simulink model "HIL_PLANT_r2025a"  (R2025a)
settings: Solver=FixedStepAuto  StartTime=0.0  StopTime=inf  MaxStep=1e-2  RelTol=1e-3  AbsTol=1e-3  EnableMultiTasking=on
undefined symbols (not defined in the file): IO334, IO336, pull, up
libraries: fl_lib x12, nesl_utility x4, speedgoatlib_fpga_analog_io x3, speedgoatlib_fpga x1
CloseFcn:
  | try,close(h1_PermanentMagnetDCMotor),end
  | clear h1_PermanentMagnetDCMotor
  | 
  | clear simlog_PermanentMagnetDCMotor
Description:
  | Permanent Magnet DC Motor
settings Model: Creator=The MathWorks, Inc.  LastModifiedBy=AEDemo
settings SolverCC: AutoScaleAbsTol=off  ConcurrentTasks=on  AlgebraicLoopSolver=TrustRegion  PositivePriorityOrder=on
settings DataIOCC: LimitDataPoints=on  SaveFormat=Array  ReturnWorkspaceOutputs=off
settings OptimizationCC: BlockReduction=off  OptimizeBlockIOStorage=off  ReuseModelBlockBuffer=off  InitFltsAndDblsToZero=on
settings DebuggingCC: SolverPrmCheckMsg=warning  TasksWithSamePriorityMsg=none  UnconnectedInputMsg=warning  UnconnectedOutputMsg=warning  UnconnectedLineMsg=warning  AllowSymbolicDim=off  PregeneratedLibrarySubsystemCodeDiagnostic=none  SFUnexpectedBacktrackingDiag=warning  SFNoUnconditionalDefaultTransitionDiag=warning  SFExecutionAtInitializationDiag=none  ArithmeticOperatorsInVariantConditions=warning
settings HardwareCC: ProdBitPerLong=64.0  ProdLongLongMode=on  ProdHWDeviceType=Intel->x86-64 (Linux 64)  TargetLongLongMode=on
settings ModelReferenceCC: EnableRefExpFcnMdlSchedulingChecks=on  PropagateSignalLabelsOutOfModel=off
settings SFSimCC: SimUseLocalCustomCode=off  CustomCodeUndefinedFunction=UseInterfaceOnly
settings RTWCC: SystemTargetFile=speedgoat.tlc  TemplateMakefile=slrealtime_default_tmf  RTWUseLocalCustomCode=off  Toolchain=Simulink Real-Time Toolchain  BuildConfiguration=Faster Runs  CodeExecutionProfiling=on  TargetLang=C++  GPUComputeCapability=3.5  DLArmComputeVersion=19.05  Description=Speedgoat Real-Time Target Machine
settings CodeAppCC: StateflowObjectComments=on
settings SimulinkRealTimeTargetCC: SLRTFileLogMaxRuns=1.0  ExtModeMaxTrigDuration=10.0  ExtModeStaticAllocSize=1000000.0  ExtModeTransport=0.0  MultiwordLength=2048.0  DynamicStringBufferSize=256.0  PreserveMATLABNamespacesInGeneratedCode=on  SubcomponentCodeInterfacePackaging=Reusable function  MATLABClassNameForMDSCustomization=Simulink.SoftwareTarget.GRTCustomization  InstructionSetFMA=off  LogToMDFFile=off
settings ConfigComp: CovMetricSettings=dw  CovSaveCumulativeToWorkspaceVar=on  CovSaveSingleToWorkspaceVar=on  CovExternalEMLEnable=off  CovSFcnEnable=off
settings SimscapeCC: SimscapeLogType=all  SimscapeLogSimulationStatistics=on  SimscapeLogName=simlog_PermanentMagnetDCMotor  SimscapeLogDataHistory=10000.0

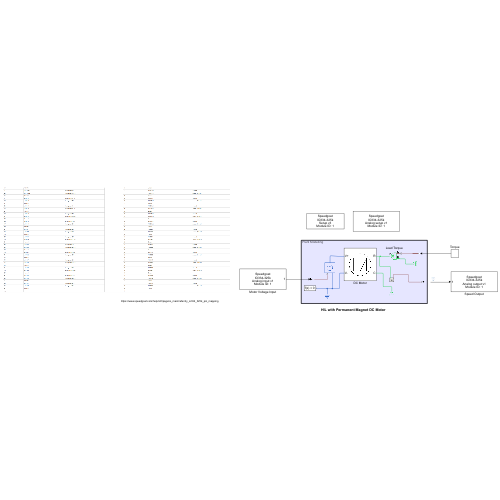
[thumbnail: Simulink's stored preview of the top-level diagram]
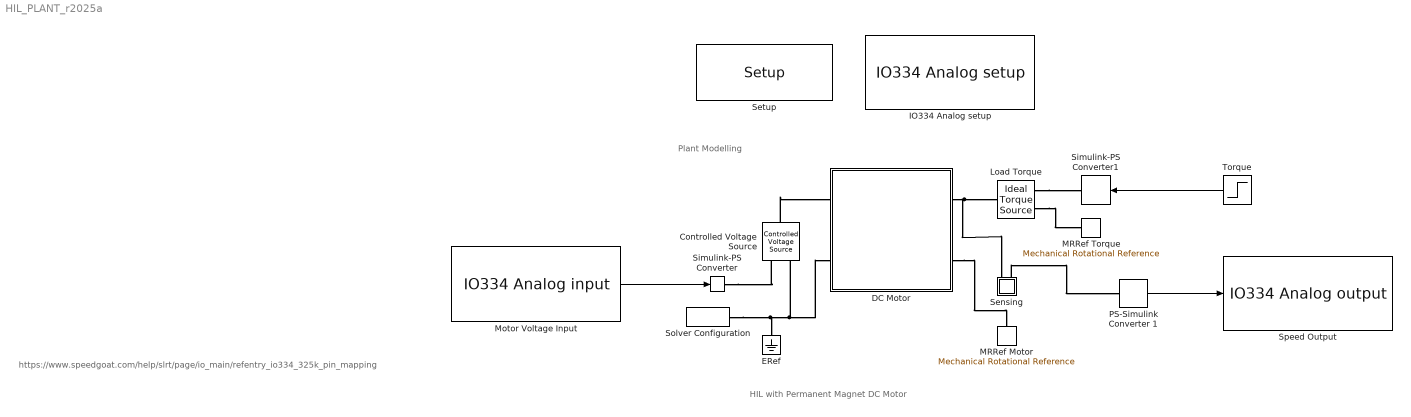
== system HIL_PLANT_r2025a ==
  note: https://www.speedgoat.com/help/slrt/page/io_main/refentry_io334_325k_pin_mapping
  note: Plant Modelling
  note: HIL with Permanent Magnet DC Motor
  Controlled Voltage Source : fl_lib/Electrical/Electrical Sources/Controlled Voltage Source
  DC Motor : Subsystem  Tag=PublishSubsystem
      mask Display:
      | % Circle, in/out, and 'M'
      | image('PermanentMagnetDCMotorMaskIcon.png');
      | 
      | % % Circle
      | % plot(sin(0:0.1:2.2*pi)*0.9,cos(0:0.1:2.2*pi)*0.9);
      | %
      | % % In/out
      | % plot([-1.3 -0.9],[0 0]);
      | % plot([1.3 0.9],[0 0]);
      | %
      | % % 'M'
      | % plot([0.5 0.5],[-0.5 0.5]);
      | % plot([-0.5 -0.5],[-0.5 0.5]);
      | % plot([0.5 0],[0.5 -0.5]);
      | % plot([-0.5 0],[0.5 -0.5]);
      | 
      | % Plot points to set plot range
      | color('white');plot(1.5,1.5);plot(-1.5,-1.5)
      | color('black');
      | 
      | port_label('RConn',1,'R');
      | port_label('RConn',2,'C');
      | port_label('LConn',1,'V+');
      | port_label('LConn',2,'V-');
  ERef : fl_lib/Electrical/Electrical Elements/Electrical Reference
  IO334 Analog setup : speedgoatlib_fpga_analog_io/IO334/IO334 Analog setup  id=1  parEnableCodeModule1=off  parEnableCodeModule2=off  parEnableCodeModule3=off  parEnableCodeModule4=off  parEnableCodeModule5=off  parEnableCodeModule6=off  parEnableCodeModule7=off  parEnableCodeModule8=off  parAdcEnableIndividualTrigger=off  parAdcDisableSampleRead=off  parAdcTriggerMode1=Model Step  parAdcSampleRate1=1e5  parAdcDioTriggerChannel1=1  parAdcInternalTrigger1=<empty>  parAdcOversampling1=None  parAdcTriggerMode2=Model Step  parAdcSampleRate2=1e5  parAdcDioTriggerChannel2=1  parAdcInternalTrigger2=<empty>  parAdcOversampling2=None  parAdcTriggerMode3=Model Step  parAdcSampleRate3=1e5  parAdcDioTriggerChannel3=1  parAdcInternalTrigger3=<empty>  parAdcOversampling3=None  parAdcTriggerMode4=Model Step  parAdcSampleRate4=1e5  parAdcDioTriggerChannel4=1  parAdcInternalTrigger4=<empty>  parAdcOversampling4=None  parAdcTriggerMode5=Model Step  parAdcSampleRate5=1e5  parAdcDioTriggerChannel5=1  parAdcInternalTrigger5=<empty>  parAdcOversampling5=None  parAdcTriggerMode6=Model Step  parAdcSampleRate6=1e5  parAdcDioTriggerChannel6=1  parAdcInternalTrigger6=<empty>  parAdcOversampling6=None  parAdcTriggerMode7=Model Step  parAdcSampleRate7=1e5  parAdcDioTriggerChannel7=1  parAdcInternalTrigger7=<empty>  parAdcOversampling7=None  parAdcTriggerMode8=Model Step  parAdcSampleRate8=1e5  parAdcDioTriggerChannel8=1  parAdcInternalTrigger8=<empty>  parAdcOversampling8=None  parAdcReadPrevValueIndividualTrigger=off  parAdcEnableFrame=off  parAdcTriggerMode=I/O Module Clock  parAdcReadPrevValue=on  parAdcSampleRate=100e3  parAdcDioTriggerChannel=1  parAdcInternalTrigger=<empty>  parAdcOversampling=None  parAdcTriggerResolution=1e-08  parAdcSampleRateFrame=1e5  parAdcFrameSize=100  parAdcSampleTime=-1  parDacTriggerMode=Model Step  parDacInternalTrigger=<empty>  parDacDioTriggerChannel=1  parDacEnableFrame=on  parDacFifoThreshold=100  parDacTriggerResolution=1e-08  parDacSampleRate=1e6  parDacFrameSize=1000  parDacSampleTime=-1  parAdcChannel1=on  parAdcChannel2=off  parAdcChannel3=off  parAdcChannel4=off  parAdcChannel5=off  parAdcChannel6=off  parAdcChannel7=off  parAdcChannel8=off  parAdcChannel9=off  parAdcChannel10=off  parAdcChannel11=off  parAdcChannel12=off  parAdcChannel13=off  parAdcChannel14=off  parAdcChannel15=off  parAdcChannel16=off  parAdcAutoCorrection=on  parDacChannel1=on  parDacChannel2=off  parDacChannel3=off  parDacChannel4=off  parDacChannel5=off  parDacChannel6=off  parDacChannel7=off  parDacChannel8=off  parDacChannel9=off  parDacChannel10=off  parDacChannel11=off  parDacChannel12=off  parDacChannel13=off  parDacChannel14=off  parDacChannel15=off  parDacChannel16=off  parDacRange1=+-2.5 V  parDacInitValue1=0  parDacReset1=on  parDacRange2=+-10 V  parDacInitValue2=0  parDacReset2=on  parDacRange3=+-5 V  parDacInitValue3=0  parDacReset3=off  parDacRange4=+-5 V  parDacInitValue4=0  parDacReset4=off  parDacRange5=+-5 V  parDacInitValue5=0  parDacReset5=off  parDacRange6=+-5 V  parDacInitValue6=0  parDacReset6=off  parDacRange7=+-5 V  parDacInitValue7=0  parDacReset7=off  parDacRange8=+-5 V  parDacInitValue8=0  parDacReset8=off  parDacRange9=+-5 V  parDacInitValue9=0  parDacReset9=off  parDacRange10=+-5 V  parDacInitValue10=0  parDacReset10=off  parDacRange11=+-5 V  parDacInitValue11=0  parDacReset11=off  parDacRange12=+-5 V  parDacInitValue12=0  parDacReset12=off  parDacRange13=+-5 V  parDacInitValue13=0  parDacReset13=off  parDacRange14=+-5 V  parDacInitValue14=0  parDacReset14=off  parDacRange15=+-5 V  parDacInitValue15=0  parDacReset15=off  parDacRange16=+-5 V  parDacInitValue16=0  parDacReset16=off  parDacAutoCorrection=on
      settings: SourceProductName=Analog IO
  Load Torque : fl_lib/Mechanical/Mechanical Sources/Ideal Torque Source
  MRRef Motor : fl_lib/Mechanical/Rotational Elements/Mechanical Rotational Reference
  MRRef Torque : fl_lib/Mechanical/Rotational Elements/Mechanical Rotational Reference
  Motor Voltage Input : speedgoatlib_fpga_analog_io/IO334/IO334 Analog input  id=1  parSampleTime=-1  pciSlot=[-1,-1]  parAiChannels=1  parAiChannelsStreamed=1  parAiReadPrevValue=0  parAiEnableFrame=0  parAdcCoupling=[1 1 1 1]  parAdcContSampling=0  parAdcDmaEnable=0  parAdcActiveDmaDevices=[1 1 1 1]  parAiFrameSize=100
      settings: SourceProductName=Analog IO
  PS-Simulink Converter 1 : nesl_utility/PS-Simulink Converter  PhysicalDomain=network_engine_domain  SubClassName=ps_output  LeftPortType=input  RightPortType=output  PseudoPeriodic=off  Frequencies=[]  VectorFormat=1-D array  Unit=rad/s  AffineConversion=off
  Sensing : Subsystem
      mask Display: disp('w');
  Setup : speedgoatlib_fpga/Setup/Setup  Parameter124={}  board=IO334-325k  id=1  pciSlot=-1  device_id=1  bitstreamFilePath=[]  bitstreamFile=Please select...  rearEnb_1=off  rearIO_1=None  rearEnb_2=off  rearIO_2=None  ProgSpiFlash=off  ProgBPIFlash=off  useFpgaDmaController=off  PullRPort15=pull-up 3.3V  PullRPort31=pull-up 3.3V  PullRPort47=pull-up 3.3V  PullRPort63=pull-up 3.3V  diffLineTermination_1=on  diffLineTermination_2=on  diffLineTermination_3=on  diffLineTermination_4=on  diffLineTermination_5=on  diffLineTermination_6=on  diffLineTermination_7=on  diffLineTermination_8=on  diffLineTermination_9=on  diffLineTermination_10=on  diffLineTermination_11=on  diffLineTermination_12=on  diffLineTermination_13=on  diffLineTermination_14=on  diffLineTermination_15=on  diffLineTermination_16=on  diffLineTermination_17=on  diffLineTermination_18=on  diffLineTermination_19=on  diffLineTermination_20=on  diffLineTermination_21=on  diffLineTermination_22=on  diffLineTermination_23=on  diffLineTermination_24=on  diffLineTermination_25=on  diffLineTermination_26=on  diffLineTermination_27=on  diffLineTermination_28=on  diffLineTermination_29=on  diffLineTermination_30=on  diffLineTermination_31=on  diffLineTermination_32=on  Vi_Pull_36x_1=Floating  Vo_36x_1=3.3V  Vi_Pull_36x_2=Floating  Vo_36x_2=3.3V  Vi_Pull_36x_3=Floating  Vo_36x_3=3.3V  Vi_Pull_36x_4=Floating  Vo_36x_4=3.3V  Vi_Pull_36x_5=Floating  Vo_36x_5=3.3V  Vi_Pull_36x_6=Floating  Vo_36x_6=3.3V  Vi_Pull_36x_7=Floating  Vo_36x_7=3.3V  Vi_Pull_36x_8=Floating  Vo_36x_8=3.3V  Vi_Pull_36x_9_16=Floating  Vo_36x_9_16=3.3V  Vi_Pull_36x_17_24=Floating  Vo_36x_17_24=3.3V  Vi_Pull_36x_25_32=Floating  Vo_36x_25_32=3.3V  Vi_Pull_36x_33_40=Floating  Vo_36x_33_40=3.3V  Vi_Pull_36x_41_48=Floating  Vo_36x_41_48=3.3V  Vi_Pull_36x_49_56=Floating  Vo_36x_49_56=3.3V  Vi_Pull_36x_57_64=Floating  Vo_36x_57_64=3.3V  PullRPort0_1=pull-up  VioPort0_1=3.3V  PullRPort1_1=pull-up  VioPort1_1=3.3V  PullRPort2_1=pull-up  VioPort2_1=3.3V  PullRPort3_1=pull-up  VioPort3_1=3.3V  PullRPort4_1=pull-up  VioPort4_1=3.3V  PullRPort5_1=pull-up  VioPort5_1=3.3V  PullRPort6_1=pull-up  VioPort6_1=3.3V  diffLineTermination_rear1_1=on  diffLineTermination_rear1_2=on  diffLineTermination_rear1_3=on  diffLineTermination_rear1_4=on  diffLineTermination_rear1_5=on  diffLineTermination_rear1_6=on  diffLineTermination_rear1_7=on  diffLineTermination_rear1_8=on  PullRPort0_2=pull-up  VioPort0_2=3.3V  PullRPort1_2=pull-up  VioPort1_2=3.3V  PullRPort2_2=pull-up  VioPort2_2=3.3V  PullRPort3_2=pull-up  VioPort3_2=3.3V  PullRPort4_2=pull-up  VioPort4_2=3.3V  PullRPort5_2=pull-up  VioPort5_2=3.3V  PullRPort6_2=pull-up  VioPort6_2=3.3V  diffLineTermination_rear2_1=on  diffLineTermination_rear2_2=on  diffLineTermination_rear2_3=on  diffLineTermination_rear2_4=on  diffLineTermination_rear2_5=on  diffLineTermination_rear2_6=on  diffLineTermination_rear2_7=on  diffLineTermination_rear2_8=on
      settings: SourceProductName=IO3xx
  Simulink-PS Converter : nesl_utility/Simulink-PS Converter  PhysicalDomain=network_engine_domain  SubClassName=ps_input  LeftPortType=input  RightPortType=output  PseudoPeriodic=off  Frequencies=[]  NoiseDistribution=none  NoiseParameters=[]  Unit=V  AffineConversion=off  FilteringAndDerivatives=provide  SimscapeFilterOrder=1  InputFilterTimeConstant=0.001  UdotUserProvided=0
  Simulink-PS Converter1 : nesl_utility/Simulink-PS Converter  PhysicalDomain=network_engine_domain  SubClassName=ps_input  LeftPortType=input  RightPortType=output  PseudoPeriodic=off  Frequencies=[]  NoiseDistribution=none  NoiseParameters=[]  Unit=1  AffineConversion=off  FilteringAndDerivatives=zero  SimscapeFilterOrder=1  InputFilterTimeConstant=.001  UdotUserProvided=0
  Solver Configuration : nesl_utility/Solver Configuration  PhysicalDomain=network_engine_domain  SubClassName=solver  LeftPortType=input  RightPortType=generic  Tones=[]  Harmonics=[]  SimulateNoise=off  Profile=off  UseLocalSampling=off  EnableSwitchedLinearOptims=on  FrequencyDomain=off  UseCCode=off  RelTol=0.001  AbsTol=1e-06  MinStep=1e-09  ToWorkspace=off  RevertToSquareIcSolve=off  NumHomotopyIterations=100  PhasorMode=off  PhasorModeNumHarmonics=1  ConsistencySolver=NEWTON_XTOL_AFTER_FTOL  IndexReductionMethod=DerivativeReplacement  DoDC=off  ResidualTolerance=1e-9  ConsistencyTolSource=GLOBAL  ConsistencyAbsTol=0.001  ConsistencyRelTol=0.001  ConsistencyTolFactor=0.001  UseLocalSolver=off  LocalSolverChoice=NE_BACKWARD_EULER_ADVANCER  ResolveIndetEquations=on  FunctionEvalNumThread=1  LocalSolverSampleTime=.001  DoFixedCost=off  MaxNonlinIter=3  MaxModeIter=2  ComputeImpulses=off  ImpulseIterations=2  LinearAlgebra=auto  LinearAlgebraNumThread=0  EquationFormulation=NE_TIME_EF  DelaysMemoryBudget=1024  AutomaticFiltering=on  FilteringTimeConstant=0.001  PartitionStorageMethod=AS_NEEDED  PartitionMemoryBudget=1024  PartitionMethod=FAST  MultibodyUseLocalSolver=on  MultibodyLocalSolverChoice=ODE1  MultibodyLocalSolverSampleTime=0.001
  Speed Output : speedgoatlib_fpga_analog_io/IO334/IO334 Analog output  id=1  parSampleTime=-1  pciSlot=[-1,-1]  board=IO336-325k  parAoChannels=1  parAoVoltageRange=3  parDacOverRange=[0 0 0 0 0 0 0 0]  parAoInitValues=0  parAoReset=1  parDacSyncOut=1  parAoEnableFrame=0  parDacActiveDmaDevices=[1 1 1 1]  parDacDmaLatency=2  parAoFrameSize=1000
      settings: SourceProductName=Analog IO
  Torque : Step  After=-0.1  SampleTime=0
  wires:
  Torque/1 -> Simulink-PS Converter1/1
  PS-Simulink Converter 1/1 -> Speed Output/1
  Motor Voltage Input/1 -> Simulink-PS Converter/1
  connections:
  Solver Configuration/RConn1 -- Controlled Voltage Source/RConn2 -- DC Motor/LConn2 -- ERef/LConn1
  Simulink-PS Converter/RConn1 -- Controlled Voltage Source/RConn1
  Controlled Voltage Source/LConn1 -- DC Motor/LConn1
  DC Motor/RConn2 -- MRRef Motor/LConn1
  DC Motor/RConn1 -- Load Torque/LConn1 -- Sensing/LConn1
  Load Torque/RConn2 -- MRRef Torque/LConn1
  Load Torque/RConn1 -- Simulink-PS Converter1/RConn1
  Sensing/LConn2 -- PS-Simulink Converter 1/LConn1

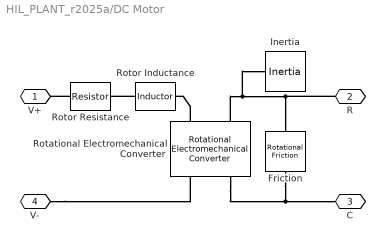
== system HIL_PLANT_r2025a/DC Motor ==
  Friction : fl_lib/Mechanical/Rotational Elements/Rotational Friction  brkwy_trq=0.002 N*m  brkwy_vel=0.1 rad/s  Col_trq=0.001 N*m  visc_coef=0.00001 N*m/(rad/s)  w_specify=off  w_priority=High  w=0 rad/s  w_nominal_specify=off  w_nominal_value=1  w_nominal_unit=rad/s  t_specify=off  t_priority=High  t=0 N*m  t_nominal_specify=off  t_nominal_value=1  t_nominal_unit=N*m
  Inertia : fl_lib/Mechanical/Rotational Elements/Inertia  inertia=0.0001 kg*m^2  num_ports=foundation.enum.numPorts2.one  w_specify=off  w_priority=High  w=0 rad/s  w_nominal_specify=off  w_nominal_value=1  w_nominal_unit=rad/s  t_specify=off  t_priority=High  t=0 N*m  t_nominal_specify=off  t_nominal_value=1  t_nominal_unit=N*m
  Rotational Electromechanical Converter : fl_lib/Electrical/Electrical Elements/Rotational Electromechanical Converter  K=0.1 V*s/rad  i_specify=off  i_priority=High  i=0 A  i_nominal_specify=off  i_nominal_value=1  i_nominal_unit=A  v_specify=off  v_priority=High  v=0 V  v_nominal_specify=off  v_nominal_value=1  v_nominal_unit=V  t_specify=off  t_priority=High  t=0 N*m  t_nominal_specify=off  t_nominal_value=1  t_nominal_unit=N*m  w_specify=off  w_priority=High  w=0 rad/s  w_nominal_specify=off  w_nominal_value=1  w_nominal_unit=rad/s
  Rotor Inductance : fl_lib/Electrical/Electrical Elements/Inductor  l=0.02 H  r=0 Ohm  g=1e-09 1/Ohm  i_specify=off  i_priority=High  i=0 A  i_nominal_specify=off  i_nominal_value=1  i_nominal_unit=A  v_specify=off  v_priority=High  v=0 V  v_nominal_specify=off  v_nominal_value=1  v_nominal_unit=V  i_L_specify=on  i_L_priority=High  i_L=0 A  i_L_nominal_specify=off  i_L_nominal_value=1  i_L_nominal_unit=A
  Rotor Resistance : fl_lib/Electrical/Electrical Elements/Resistor  Tag=Factory Generic  R=1.5 Ohm  i_specify=off  i_priority=High  i=0 A  i_nominal_specify=off  i_nominal_value=1  i_nominal_unit=A  v_specify=off  v_priority=High  v=0 V  v_nominal_specify=off  v_nominal_value=1  v_nominal_unit=V
  V+ : PMIOPort  Side=Left
  R : PMIOPort  Port=2  Side=Right
  C : PMIOPort  Port=3  Side=Right
  V- : PMIOPort  Port=4  Side=Left
  connections:
  Rotational Electromechanical Converter/LConn1 -- Rotor Inductance/RConn1
  V-/RConn1 -- Rotational Electromechanical Converter/RConn1
  Rotor Resistance/LConn1 -- V+/RConn1
  Rotor Inductance/LConn1 -- Rotor Resistance/RConn1
  Rotational Electromechanical Converter/LConn2 -- R/RConn1 -- Friction/LConn1 -- Inertia/LConn1
  Rotational Electromechanical Converter/RConn2 -- C/RConn1 -- Friction/RConn1

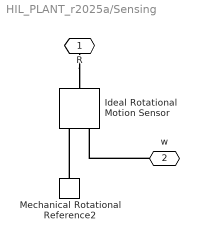
== system HIL_PLANT_r2025a/Sensing ==
  Ideal Rotational Motion Sensor : fl_lib/Mechanical/Mechanical Sensors/Ideal Rotational Motion Sensor  reference=foundation.enum.MeasurementReference.difference  acceleration_port=false  velocity_port=true  position_port=false  wrap_angle=simscape.enum.onoff.off  offset=0 rad
      settings: InternalSimscapePortConfiguration="{\"Bottom\":[],\"Left\":[{\"id\":\"R\",\"label\":\"R\",\"type\":\"foundation.mechanical.rotational.rotational\"}],\"Right\":[{\"id\":\"C\",\"label\":\"C\",\"type\":\"foundation.mechanical.rotational.rotational\"},{\"id\":\"W\",\"label\":\"W\",\"type\":\"output\"}],\"Top\":[]}"
  Mechanical Rotational Reference2 : fl_lib/Mechanical/Rotational Elements/Mechanical Rotational Reference
  R : PMIOPort  Side=Left
  w : PMIOPort  Port=2  Side=Left
  connections:
  w/RConn1 -- Ideal Rotational Motion Sensor/RConn2
  R/RConn1 -- Ideal Rotational Motion Sensor/LConn1
  Mechanical Rotational Reference2/LConn1 -- Ideal Rotational Motion Sensor/RConn1
